simulink model "Assembly"  (R2013a)
settings: Solver=ode45  StartTime=0.0  StopTime=inf  RelTol=1e-3
undefined symbols (not defined in the file): Base_Assembly, Sub_Assembly1, Sub_Assembly2, Sub_Assembly3, Sub_Assembly4
libraries: mblibv1 x18
settings Model: Creator=Samvrit  LastModifiedBy=Samvrit
settings SimMechanicsCC: VisOnUpdateDiagram=on  VisDuringSimulation=on

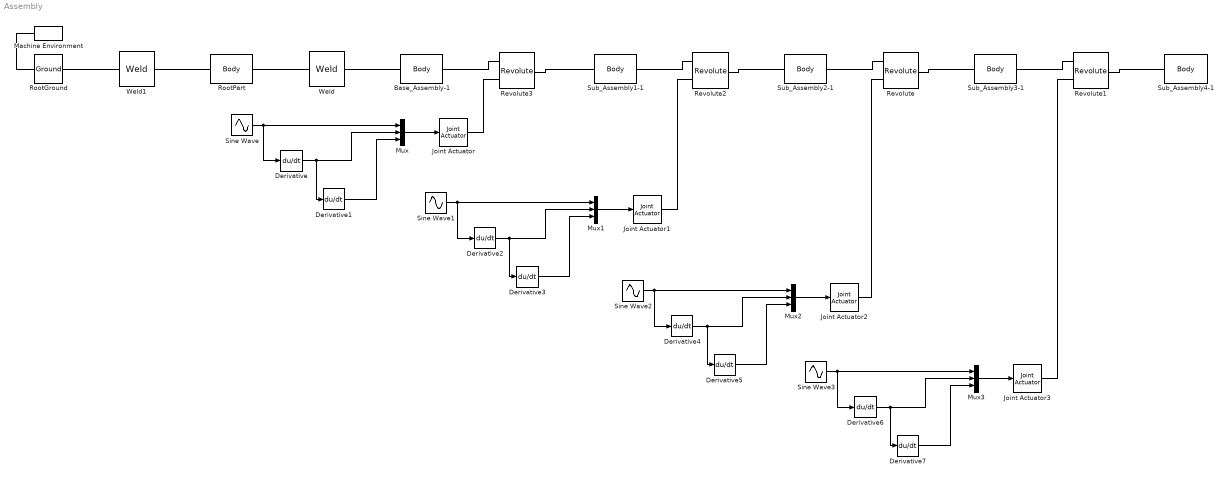
== system Assembly ==
  Base_Assembly-1 : mblibv1/Bodies/Body  LConnTagsString=CS2  RConnTagsString=CS3  UpdateFromCAD=on  PMImportedID=Base_Assembly-1  DialogClass=MechanicalBodyBlock  Mass=0.816132  MassUnits=kg  InertiaUnits=kg*m^2  Inertia=[0.00101868,2.68456e-14,-0.000208027;2.68456e-14,0.00141452,-5.88219e-14;-0.000208027,-5.88219e-14,0.000763124]  Shape=Cylinder  ShapeDims=[1 1]  ShapeUnits=m  ShapeUse=false  Density=1  DensityUnits=kg/m^3  DensityUse=false  GraphicsMode=GFXFILE  GraphicsFileName=Assembly - Base_Assembly-1.STL  BodyColorSelMode=COLORPALETTE  BodyColor=[0;0;1]  AttachedToCS=CS1  CG=Right$CG$[0.0863608 0.0666392 0.155753]$WORLD$WORLD$m$[1 0 0;0 1 0;0 0 1]$3x3 Transform$rad$WORLD$false$Base_Assembly-1::CG(AUTOGEN)  WorkingFrames=Right$CS1$[-0.0257981 -0.00724452 0.107815]$WORLD$WORLD$m$[1 0 0;0 1 0;0 0 1]$3x3 Transform$rad$WORLD$false$Base_Assembly-1::CS1(AUTOGEN)#Left$CS2$[0.0863608 0.0666392 0.155753]$WORLD$WORLD$m$[1 0 0;0 1 0;0 0 1]$3x3 Transform$rad$WORLD$true$Assembly/RootPart:-:Base_Assembly-1::Base_Assembly-1(AUTOGEN)#Right$CS3$[0.0918311 0.0666392 0.120815]$WORLD$WORLD$m$[1 0 0;0 1 0;0 0 1]$3x3 Transform$rad$WORLD$true$Base_Assembly-1:-:Sub_Assembly1-1::Base_Assembly-1(AUTOGEN)  CGPos=[0.0863608 0.0666392 0.155753]  CGRot=[1 0 0;0 1 0;0 0 1]  CS0Pos=[]  CS0Rot=[]  CS1Pos=[-0.0257981 -0.00724452 0.107815]  CS1Rot=[1 0 0;0 1 0;0 0 1]  CS2Pos=[0.0863608 0.0666392 0.155753]  CS2Rot=[1 0 0;0 1 0;0 0 1]  CS3Pos=[0.0918311 0.0666392 0.120815]  CS3Rot=[1 0 0;0 1 0;0 0 1]  CS4Pos=[]  CS4Rot=[]  CS5Pos=[]  CS5Rot=[]  CS6Pos=[]  CS6Rot=[]  CS7Pos=[]  CS7Rot=[]  CS8Pos=[]  CS8Rot=[]  CS9Pos=[]  CS9Rot=[]  CS10Pos=[]  CS10Rot=[]  CS11Pos=[]  CS11Rot=[]  CS12Pos=[]  CS12Rot=[]  CS13Pos=[]  CS13Rot=[]  CS14Pos=[]  CS14Rot=[]  CS15Pos=[]  CS15Rot=[]  CS16Pos=[]  CS16Rot=[]  CS17Pos=[]  CS17Rot=[]  CS18Pos=[]  CS18Rot=[]  CS19Pos=[]  CS19Rot=[]  CS20Pos=[]  CS20Rot=[]
  Derivative{,1..7} (8 alike) : Derivative
  Joint Actuator{,1..3} (4 alike) : mblibv1/Sensors &  Actuators/Joint Actuator  UpdateFromCAD=off  PhysicalDomain=Mechanical  PortType=blob  ActuationStyle=Motion  AngleUnits=deg  ArcVelocityUnits=deg/s  ArcAccelerationUnits=deg/s^2  CoordPositionUnits=m  VelocityUnits=m/s  AccelerationUnits=m/s^2  ForceUnits=N  TorqueUnits=N*m  ActiveIO=on  Width=3  DialogClass=MechanicalActuatorBlock  Primitive=R1  ReferenceFrame=Absolute (World)
  Machine Environment : mblibv1/Bodies/Machine Environment  PortType=env  PhysicalDomain=Mechanical  DialogTemplateClass=MECH.MachineEnvironment  SyncWhenCopied=off  Gravity=[0 -9.81 0]  GravityUnits=m/s^2  GravityAsSignal=off  Dimensionality=Auto-detect  AnalysisType=Forward dynamics  LinearAssemblyTolerance=1e-3  LinearAssemblyToleranceUnits=m  AngularAssemblyTolerance=1e-3  AngularAssemblyToleranceUnits=rad  ConstraintSolverType=Stabilizing  ConstraintRelTolerance=1e-4  ConstraintAbsTolerance=1e-4  UseRobustSingularityHandling=off  RedundancyAnalysisToleranceType=Automatically select tolerance  RedundancyAnalysisTolerance=1e-14  StatePerturbationType=Fixed  PerturbationSize=1e-5  VisualizeMachine=on  BodyVisualizationType=Use model default body geometries  BodyColorSelMode=Use model default  DefaultBodyColor=[1 0 0]
  Mux{,1..3} (4 alike) : Mux  Inputs=3
  Revolute : mblibv1/Joints/Revolute  LConnTagsString=__newl0|SA1  RConnTagsString=__newr0  UpdateFromCAD=on  PMImportedID=Sub_Assembly2-1:-:Sub_Assembly3-1  NumSAPorts=1  CutJoint=off  MarkAsCut=off  Primitives=prismatic  PrimitiveProps=R1$World$[0,0,-1]$revolute  DialogClass=JointBlock  R1Axis=[0,0,-1]
  Revolute1 : mblibv1/Joints/Revolute  LConnTagsString=__newl0|SA1  RConnTagsString=__newr0  UpdateFromCAD=on  PMImportedID=Sub_Assembly3-1:-:Sub_Assembly4-1  NumSAPorts=1  CutJoint=off  MarkAsCut=off  Primitives=prismatic  PrimitiveProps=R1$World$[0,1,0]$revolute  DialogClass=JointBlock  R1Axis=[0,1,0]
  Revolute2 : mblibv1/Joints/Revolute  LConnTagsString=__newl0|SA1  RConnTagsString=__newr0  UpdateFromCAD=on  PMImportedID=Sub_Assembly1-1:-:Sub_Assembly2-1  NumSAPorts=1  CutJoint=off  MarkAsCut=off  Primitives=prismatic  PrimitiveProps=R1$World$[1,0,0]$revolute  DialogClass=JointBlock  R1Axis=[1,0,0]
  Revolute3 : mblibv1/Joints/Revolute  LConnTagsString=__newl0|SA1  RConnTagsString=__newr0  UpdateFromCAD=on  PMImportedID=Base_Assembly-1:-:Sub_Assembly1-1  NumSAPorts=1  CutJoint=off  MarkAsCut=off  Primitives=prismatic  PrimitiveProps=R1$World$[0,0,-1]$revolute  DialogClass=JointBlock  R1Axis=[0,0,-1]
  RootGround : mblibv1/Bodies/Ground  UpdateFromCAD=on  PMImportedID=RootGround  LeftPortType=env  RightPortType=workingframe  PhysicalDomain=Mechanical  DialogClass=GroundBlock  CoordPosition=[0.108255,0.0656856,-0.00842688]  CoordPositionUnits=m  StateVectorMgrId=0  MachineId=[1 0]  ShowEnvPort=on
  RootPart : mblibv1/Bodies/Body  LConnTagsString=CS3  RConnTagsString=CS2  UpdateFromCAD=on  PMImportedID=Assembly/RootPart  DialogClass=MechanicalBodyBlock  Mass=0  MassUnits=kg  InertiaUnits=kg*m^2  Inertia=[0,0,0;0,0,0;0,0,0]  Shape=Cylinder  ShapeDims=[1 1]  ShapeUnits=m  ShapeUse=false  Density=1  DensityUnits=kg/m^3  DensityUse=false  GraphicsMode=MACHINE_DEFAULT  BodyColorSelMode=MACHINE_DEFAULT  BodyColor=[1;0;0]  AttachedToCS=CS1  CG=Right$CG$[0.108255 0.0656856 -0.00842688]$WORLD$WORLD$m$[1 0 0;0 1 0;0 0 1]$3x3 Transform$rad$WORLD$false$Assembly/RootPart::CG(AUTOGEN)  WorkingFrames=Right$CS1$[0 0 0]$WORLD$WORLD$m$[1 0 0;0 1 0;0 0 1]$3x3 Transform$rad$WORLD$false$Assembly/RootPart::CS1(AUTOGEN)#Right$CS2$[0.0863608 0.0666392 0.155753]$WORLD$WORLD$m$[1 0 0;0 1 0;0 0 1]$3x3 Transform$rad$WORLD$true$Assembly/RootPart:-:Base_Assembly-1::Assembly/RootPart(AUTOGEN)#Left$CS3$[0.108255 0.0656856 -0.00842688]$WORLD$WORLD$m$[1 0 0;0 1 0;0 0 1]$3x3 Transform$rad$WORLD$true$Assembly/RootPart:-:RootGround::Assembly/RootPart(AUTOGEN)  CGPos=[0.108255 0.0656856 -0.00842688]  CGRot=[1 0 0;0 1 0;0 0 1]  CS0Pos=[]  CS0Rot=[]  CS1Pos=[0 0 0]  CS1Rot=[1 0 0;0 1 0;0 0 1]  CS2Pos=[0.0863608 0.0666392 0.155753]  CS2Rot=[1 0 0;0 1 0;0 0 1]  CS3Pos=[0.108255 0.0656856 -0.00842688]  CS3Rot=[1 0 0;0 1 0;0 0 1]  CS4Pos=[]  CS4Rot=[]  CS5Pos=[]  CS5Rot=[]  CS6Pos=[]  CS6Rot=[]  CS7Pos=[]  CS7Rot=[]  CS8Pos=[]  CS8Rot=[]  CS9Pos=[]  CS9Rot=[]  CS10Pos=[]  CS10Rot=[]  CS11Pos=[]  CS11Rot=[]  CS12Pos=[]  CS12Rot=[]  CS13Pos=[]  CS13Rot=[]  CS14Pos=[]  CS14Rot=[]  CS15Pos=[]  CS15Rot=[]  CS16Pos=[]  CS16Rot=[]  CS17Pos=[]  CS17Rot=[]  CS18Pos=[]  CS18Rot=[]  CS19Pos=[]  CS19Rot=[]  CS20Pos=[]  CS20Rot=[]
  Sine Wave{,1..3} (4 alike) : Sin  Amplitude=45  SampleTime=0
  Sub_Assembly1-1 : mblibv1/Bodies/Body  LConnTagsString=CS3  RConnTagsString=CS2  UpdateFromCAD=on  PMImportedID=Sub_Assembly1-1  DialogClass=MechanicalBodyBlock  Mass=0.850196  MassUnits=kg  InertiaUnits=kg*m^2  Inertia=[0.000429886,2.65004e-07,7.38865e-06;2.65004e-07,0.0010883,-4.75425e-08;7.38865e-06,-4.75425e-08,0.00103792]  Shape=Cylinder  ShapeDims=[1 1]  ShapeUnits=m  ShapeUse=false  Density=1  DensityUnits=kg/m^3  DensityUse=false  GraphicsMode=GFXFILE  GraphicsFileName=Assembly - Sub_Assembly1-1.STL  BodyColorSelMode=COLORPALETTE  BodyColor=[0;1;0]  AttachedToCS=CS1  CG=Right$CG$[0.0944723 0.0666171 0.061243]$WORLD$WORLD$m$[1 0 0;0 1 0;0 0 1]$3x3 Transform$rad$WORLD$false$Sub_Assembly1-1::CG(AUTOGEN)  WorkingFrames=Right$CS1$[0.0758841 0.047428 0.0750282]$WORLD$WORLD$m$[1 0 0;0 1 0;0 0 1]$3x3 Transform$rad$WORLD$false$Sub_Assembly1-1::CS1(AUTOGEN)#Right$CS2$[0.134581 0.0666392 0.0587152]$WORLD$WORLD$m$[1 0 0;0 1 0;0 0 1]$3x3 Transform$rad$WORLD$true$Sub_Assembly1-1:-:Sub_Assembly2-1::Sub_Assembly1-1(AUTOGEN)#Left$CS3$[0.0918311 0.0666392 0.120815]$WORLD$WORLD$m$[1 0 0;0 1 0;0 0 1]$3x3 Transform$rad$WORLD$true$Base_Assembly-1:-:Sub_Assembly1-1::Sub_Assembly1-1(AUTOGEN)  CGPos=[0.0944723 0.0666171 0.061243]  CGRot=[1 0 0;0 1 0;0 0 1]  CS0Pos=[]  CS0Rot=[]  CS1Pos=[0.0758841 0.047428 0.0750282]  CS1Rot=[1 0 0;0 1 0;0 0 1]  CS2Pos=[0.134581 0.0666392 0.0587152]  CS2Rot=[1 0 0;0 1 0;0 0 1]  CS3Pos=[0.0918311 0.0666392 0.120815]  CS3Rot=[1 0 0;0 1 0;0 0 1]  CS4Pos=[]  CS4Rot=[]  CS5Pos=[]  CS5Rot=[]  CS6Pos=[]  CS6Rot=[]  CS7Pos=[]  CS7Rot=[]  CS8Pos=[]  CS8Rot=[]  CS9Pos=[]  CS9Rot=[]  CS10Pos=[]  CS10Rot=[]  CS11Pos=[]  CS11Rot=[]  CS12Pos=[]  CS12Rot=[]  CS13Pos=[]  CS13Rot=[]  CS14Pos=[]  CS14Rot=[]  CS15Pos=[]  CS15Rot=[]  CS16Pos=[]  CS16Rot=[]  CS17Pos=[]  CS17Rot=[]  CS18Pos=[]  CS18Rot=[]  CS19Pos=[]  CS19Rot=[]  CS20Pos=[]  CS20Rot=[]
  Sub_Assembly2-1 : mblibv1/Bodies/Body  LConnTagsString=CS3  RConnTagsString=CS2  UpdateFromCAD=on  PMImportedID=Sub_Assembly2-1  DialogClass=MechanicalBodyBlock  Mass=0.955246  MassUnits=kg  InertiaUnits=kg*m^2  Inertia=[0.000813069,2.47935e-07,-8.81681e-05;2.47935e-07,0.00189612,-9.90122e-09;-8.81681e-05,-9.90122e-09,0.00152266]  Shape=Cylinder  ShapeDims=[1 1]  ShapeUnits=m  ShapeUse=false  Density=1  DensityUnits=kg/m^3  DensityUse=false  GraphicsMode=GFXFILE  GraphicsFileName=Assembly - Sub_Assembly2-1.STL  BodyColorSelMode=COLORPALETTE  BodyColor=[1;1;0]  AttachedToCS=CS1  CG=Right$CG$[0.0951659 0.0666308 -0.0315029]$WORLD$WORLD$m$[0 0 -1;0 -1 0;-1 0 0]$3x3 Transform$rad$WORLD$false$Sub_Assembly2-1::CG(AUTOGEN)  WorkingFrames=Right$CS1$[0.180947 0.0857083 0.0737485]$WORLD$WORLD$m$[0 0 -1;0 -1 0;-1 0 0]$3x3 Transform$rad$WORLD$false$Sub_Assembly2-1::CS1(AUTOGEN)#Right$CS2$[0.0939311 0.0666392 -0.0770839]$WORLD$WORLD$m$[1 0 0;0 1 0;0 0 1]$3x3 Transform$rad$WORLD$true$Sub_Assembly2-1:-:Sub_Assembly3-1::Sub_Assembly2-1(AUTOGEN)#Left$CS3$[0.134581 0.0666392 0.0587152]$WORLD$WORLD$m$[1 0 0;0 1 0;0 0 1]$3x3 Transform$rad$WORLD$true$Sub_Assembly1-1:-:Sub_Assembly2-1::Sub_Assembly2-1(AUTOGEN)  CGPos=[0.0951659 0.0666308 -0.0315029]  CGRot=[0 0 -1;0 -1 0;-1 0 0]  CS0Pos=[]  CS0Rot=[]  CS1Pos=[0.180947 0.0857083 0.0737485]  CS1Rot=[0 0 -1;0 -1 0;-1 0 0]  CS2Pos=[0.0939311 0.0666392 -0.0770839]  CS2Rot=[1 0 0;0 1 0;0 0 1]  CS3Pos=[0.134581 0.0666392 0.0587152]  CS3Rot=[1 0 0;0 1 0;0 0 1]  CS4Pos=[]  CS4Rot=[]  CS5Pos=[]  CS5Rot=[]  CS6Pos=[]  CS6Rot=[]  CS7Pos=[]  CS7Rot=[]  CS8Pos=[]  CS8Rot=[]  CS9Pos=[]  CS9Rot=[]  CS10Pos=[]  CS10Rot=[]  CS11Pos=[]  CS11Rot=[]  CS12Pos=[]  CS12Rot=[]  CS13Pos=[]  CS13Rot=[]  CS14Pos=[]  CS14Rot=[]  CS15Pos=[]  CS15Rot=[]  CS16Pos=[]  CS16Rot=[]  CS17Pos=[]  CS17Rot=[]  CS18Pos=[]  CS18Rot=[]  CS19Pos=[]  CS19Rot=[]  CS20Pos=[]  CS20Rot=[]
  Sub_Assembly3-1 : mblibv1/Bodies/Body  LConnTagsString=CS2  RConnTagsString=CS3  UpdateFromCAD=on  PMImportedID=Sub_Assembly3-1  DialogClass=MechanicalBodyBlock  Mass=1.1576  MassUnits=kg  InertiaUnits=kg*m^2  Inertia=[0.00518587,0.000358971,0.00133807;0.000358971,0.00541515,-0.000899224;0.00133807,-0.000899224,0.00332016]  Shape=Cylinder  ShapeDims=[1 1]  ShapeUnits=m  ShapeUse=false  Density=1  DensityUnits=kg/m^3  DensityUse=false  GraphicsMode=GFXFILE  GraphicsFileName=Assembly - Sub_Assembly3-1.STL  BodyColorSelMode=COLORPALETTE  BodyColor=[0.909804;0.443137;0.0313725]  AttachedToCS=CS1  CG=Right$CG$[0.148009 0.0629405 -0.0652875]$WORLD$WORLD$m$[-0.866025 0.5 0;-0.5 -0.866025 0;0 0 1]$3x3 Transform$rad$WORLD$false$Sub_Assembly3-1::CG(AUTOGEN)  WorkingFrames=Right$CS1$[0.100495 0.0912165 -0.122623]$WORLD$WORLD$m$[-0.866025 0.5 0;-0.5 -0.866025 0;0 0 1]$3x3 Transform$rad$WORLD$false$Sub_Assembly3-1::CS1(AUTOGEN)#Left$CS2$[0.0939311 0.0666392 -0.0770839]$WORLD$WORLD$m$[1 0 0;0 1 0;0 0 1]$3x3 Transform$rad$WORLD$true$Sub_Assembly2-1:-:Sub_Assembly3-1::Sub_Assembly3-1(AUTOGEN)#Right$CS3$[0.0939311 0.109639 -0.230684]$WORLD$WORLD$m$[1 0 0;0 1 0;0 0 1]$3x3 Transform$rad$WORLD$true$Sub_Assembly3-1:-:Sub_Assembly4-1::Sub_Assembly3-1(AUTOGEN)  CGPos=[0.148009 0.0629405 -0.0652875]  CGRot=[-0.866025 0.5 0;-0.5 -0.866025 0;0 0 1]  CS0Pos=[]  CS0Rot=[]  CS1Pos=[0.100495 0.0912165 -0.122623]  CS1Rot=[-0.866025 0.5 0;-0.5 -0.866025 0;0 0 1]  CS2Pos=[0.0939311 0.0666392 -0.0770839]  CS2Rot=[1 0 0;0 1 0;0 0 1]  CS3Pos=[0.0939311 0.109639 -0.230684]  CS3Rot=[1 0 0;0 1 0;0 0 1]  CS4Pos=[]  CS4Rot=[]  CS5Pos=[]  CS5Rot=[]  CS6Pos=[]  CS6Rot=[]  CS7Pos=[]  CS7Rot=[]  CS8Pos=[]  CS8Rot=[]  CS9Pos=[]  CS9Rot=[]  CS10Pos=[]  CS10Rot=[]  CS11Pos=[]  CS11Rot=[]  CS12Pos=[]  CS12Rot=[]  CS13Pos=[]  CS13Rot=[]  CS14Pos=[]  CS14Rot=[]  CS15Pos=[]  CS15Rot=[]  CS16Pos=[]  CS16Rot=[]  CS17Pos=[]  CS17Rot=[]  CS18Pos=[]  CS18Rot=[]  CS19Pos=[]  CS19Rot=[]  CS20Pos=[]  CS20Rot=[]
  Sub_Assembly4-1 : mblibv1/Bodies/Body  LConnTagsString=CS2  UpdateFromCAD=on  PMImportedID=Sub_Assembly4-1  DialogClass=MechanicalBodyBlock  Mass=0.274259  MassUnits=kg  InertiaUnits=kg*m^2  Inertia=[0.00239407,-3.61918e-09,1.62879e-09;-3.61918e-09,0.000217632,9.3932e-05;1.62879e-09,9.3932e-05,0.00235245]  Shape=Cylinder  ShapeDims=[1 1]  ShapeUnits=m  ShapeUse=false  Density=1  DensityUnits=kg/m^3  DensityUse=false  GraphicsMode=GFXFILE  GraphicsFileName=Assembly - Sub_Assembly4-1.STL  BodyColorSelMode=COLORPALETTE  BodyColor=[1;0;0]  AttachedToCS=CS1  CG=Right$CG$[0.093931 0.0682545 -0.39259]$WORLD$WORLD$m$[1 0 0;0 0 1;0 -1 0]$3x3 Transform$rad$WORLD$false$Sub_Assembly4-1::CG(AUTOGEN)  WorkingFrames=Right$CS1$[0.0385874 -0.0559867 -0.149356]$WORLD$WORLD$m$[1 0 0;0 0 1;0 -1 0]$3x3 Transform$rad$WORLD$false$Sub_Assembly4-1::CS1(AUTOGEN)#Left$CS2$[0.0939311 0.109639 -0.230684]$WORLD$WORLD$m$[1 0 0;0 1 0;0 0 1]$3x3 Transform$rad$WORLD$true$Sub_Assembly3-1:-:Sub_Assembly4-1::Sub_Assembly4-1(AUTOGEN)  CGPos=[0.093931 0.0682545 -0.39259]  CGRot=[1 0 0;0 0 1;0 -1 0]  CS0Pos=[]  CS0Rot=[]  CS1Pos=[0.0385874 -0.0559867 -0.149356]  CS1Rot=[1 0 0;0 0 1;0 -1 0]  CS2Pos=[0.0939311 0.109639 -0.230684]  CS2Rot=[1 0 0;0 1 0;0 0 1]  CS3Pos=[]  CS3Rot=[]  CS4Pos=[]  CS4Rot=[]  CS5Pos=[]  CS5Rot=[]  CS6Pos=[]  CS6Rot=[]  CS7Pos=[]  CS7Rot=[]  CS8Pos=[]  CS8Rot=[]  CS9Pos=[]  CS9Rot=[]  CS10Pos=[]  CS10Rot=[]  CS11Pos=[]  CS11Rot=[]  CS12Pos=[]  CS12Rot=[]  CS13Pos=[]  CS13Rot=[]  CS14Pos=[]  CS14Rot=[]  CS15Pos=[]  CS15Rot=[]  CS16Pos=[]  CS16Rot=[]  CS17Pos=[]  CS17Rot=[]  CS18Pos=[]  CS18Rot=[]  CS19Pos=[]  CS19Rot=[]  CS20Pos=[]  CS20Rot=[]
  Weld : mblibv1/Joints/Weld  LConnTagsString=__newl0  RConnTagsString=__newr0  UpdateFromCAD=on  PMImportedID=Assembly/RootPart:-:Base_Assembly-1  NumSAPorts=0  CutJoint=off  MarkAsCut=off  Primitives=weld  PrimitiveProps=W$WORLD$[0.57735,0.57735,0.57735]$weld  DialogClass=JointBlock  WAxis=[0.57735,0.57735,0.57735]
  Weld1 : mblibv1/Joints/Weld  LConnTagsString=__newl0  RConnTagsString=__newr0  UpdateFromCAD=on  PMImportedID=Assembly/RootPart:-:RootGround  NumSAPorts=0  CutJoint=off  MarkAsCut=off  Primitives=weld  PrimitiveProps=W$WORLD$[0.57735,0.57735,0.57735]$weld  DialogClass=JointBlock  WAxis=[0.57735,0.57735,0.57735]
  wires:
  Mux/1 -> Joint Actuator/1
  Sine Wave/1 -> Derivative/1, Mux/1
  Derivative/1 -> Derivative1/1, Mux/2
  Derivative1/1 -> Mux/3
  Mux1/1 -> Joint Actuator1/1
  Sine Wave1/1 -> Mux1/1, Derivative2/1
  Derivative2/1 -> Mux1/2, Derivative3/1
  Derivative3/1 -> Mux1/3
  Mux2/1 -> Joint Actuator2/1
  Sine Wave2/1 -> Derivative4/1, Mux2/1
  Derivative4/1 -> Derivative5/1, Mux2/2
  Derivative5/1 -> Mux2/3
  Mux3/1 -> Joint Actuator3/1
  Sine Wave3/1 -> Mux3/1, Derivative6/1
  Derivative6/1 -> Mux3/2, Derivative7/1
  Derivative7/1 -> Mux3/3
  connections:
  RootPart/RConn1 -- Weld/LConn1
  Weld/RConn1 -- Base_Assembly-1/LConn1
  Sub_Assembly2-1/RConn1 -- Revolute/LConn1
  Revolute/RConn1 -- Sub_Assembly3-1/LConn1
  Sub_Assembly3-1/RConn1 -- Revolute1/LConn1
  Revolute1/RConn1 -- Sub_Assembly4-1/LConn1
  Sub_Assembly1-1/RConn1 -- Revolute2/LConn1
  Revolute2/RConn1 -- Sub_Assembly2-1/LConn1
  Base_Assembly-1/RConn1 -- Revolute3/LConn1
  Revolute3/RConn1 -- Sub_Assembly1-1/LConn1
  RootGround/RConn1 -- Weld1/LConn1
  Weld1/RConn1 -- RootPart/LConn1
  RootGround/LConn1 -- Machine Environment/RConn1
  Joint Actuator/RConn1 -- Revolute3/LConn2
  Joint Actuator1/RConn1 -- Revolute2/LConn2
  Joint Actuator2/RConn1 -- Revolute/LConn2
  Joint Actuator3/RConn1 -- Revolute1/LConn2
